simulink model "surveillance"  (Simulink 6.5)
settings: Solver=VariableStepDiscrete  StartTime=0.0  StopTime=inf  RelTol=1e-3
undefined symbols (not defined in the file or in its folder): gray
libraries: dspsnks4 x2, dspobslib x2, dspmtrx3 x2, dspsrcs4 x1, dspwin32 x1
settings Model: Creator=jacobf  LastModifiedBy=JacobF

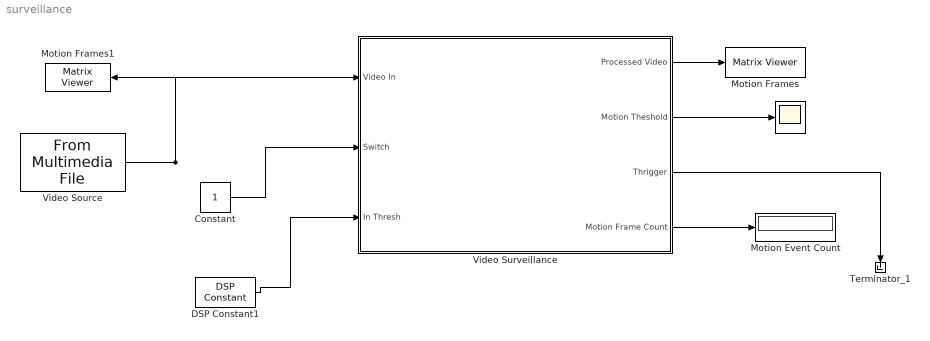
== system surveillance ==
  " " : Scope
      settings: TimeRange=18  YMin=0  YMax=500000
  Constant : Constant  Value=1  OutDataType=sfix(16)  ConRadixGroup=Use specified scaling  OutScaling=2^0  SampleTime=inf  FramePeriod=inf
  DSP Constant1 : dspsrcs4/DSP Constant  SystemSampleTime=-1  Value=1.5e5  SampleMode=Discrete  discreteOutput=Sample-based  continuousOutput=Sample-based  sampTime=1/15  framePeriod=2  dataType=int32  isSigned=on  wordLen=16  udDataType=sfix(16)  fracBitsMode=Best precision  numFracBits=15  InterpretAs1D=-inf  Ts=-inf  FramebasedOutput=-inf
      settings: additionalParams=on
  Motion Event Count : Display
  Motion Frames : dspsnks4/Matrix Viewer  DialogController=dspdialog.MatrixViewer  DialogControllerArgs=DataTag0  ImageParams=off  CMapStr=gray(256)  AxisColorbar=off  AxisParams=off  AxisOrigin=Upper left corner  XLabel=X-axis  YLabel=Y-axis  ZLabel=Z-axis  FigPos=[326 381 283 245]  AxisZoom=on
      settings: YMin=0  YMax=255
  Motion Frames1 : dspsnks4/Matrix Viewer  Orientation=left  DialogController=dspdialog.MatrixViewer  DialogControllerArgs=DataTag1  ImageParams=off  CMapStr=gray(256)  AxisColorbar=off  AxisParams=off  AxisOrigin=Upper left corner  XLabel=X-axis  YLabel=Y-axis  ZLabel=Z-axis  FigPos=[39 384 279 242]  AxisZoom=on
      settings: YMin=0  YMax=255
  Terminator_1 : Terminator
      settings: Orientation=down
  Video Source : dspwin32/From Multimedia File  DialogController=dspDDGCreate  DialogControllerArgs=DataTag2  inputFilename=vipmen.avi  loop=on  numPlays=inf  outputStreams=Video and audio  videoDataType=uint8  audioDataType=int16  inheritSampleTime=on  userDefinedSampleTime=1/30  noAudioOutput=off  isIntensityVideo=on  outputEOF=off
  "Video Surveillance " : Subsystem
  wires:
  Video Source/1 -> Motion Frames1/1, "Video Surveillance "/1(Video In)
  "Video Surveillance "/1(Processed Video) -> Motion Frames/1
  "Video Surveillance "/4(Motion Frame Count) -> Motion Event Count/1
  Constant/1 -> "Video Surveillance "/2(Switch)
  "Video Surveillance "/2(Motion Theshold) -> " "/1
  DSP Constant1/1 -> "Video Surveillance "/3(In Thresh)
  "Video Surveillance "/3(Thrigger) -> Terminator_1/1

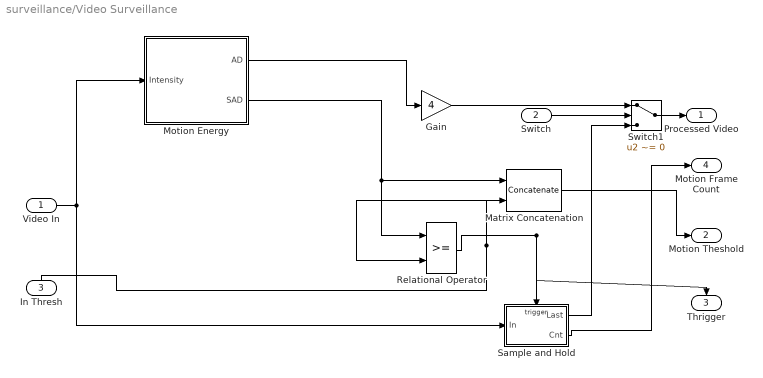
== system surveillance/Video Surveillance  ==
  Video In : Inport
  Switch : Inport  Port=2
  In Thresh : Inport  Orientation=up  Port=3
  Gain : Gain  Gain=4  ParameterDataType=uint(8)  OutDataTypeMode=Specify via dialog  OutDataType=uint(8)  SaturateOnIntegerOverflow=on
  Matrix Concatenation : Concatenate  Mode=Vertical matrix concatenation
  Motion Energy : Subsystem
  Relational Operator : RelationalOperator  LogicOutDataTypeMode=Boolean  InputSameDT=on
  Sample and Hold : Subsystem  AncestorBlock=dspsigops/Sample and Hold  TreatAsAtomicUnit=on  mask(Sample and Hold){trig=Either edge, initCond=0}
      mask prompts: trig "Trigger type:"; initCond "Initial condition:"
      mask help: Sample and hold input signal.
      mask init:
      | switch trig
      | case 1, s='rising';
      | case 2, s='falling';
      | case 3, s='either';
      | end
      | set_param([gcb '/Trigger'],'triggertype',s);
      mask Help: web(dspbhelp);
      mask StyleString: popup(Rising edge|Falling edge|Either edge),edit
      mask Display: disp('S/H')
  Switch1 : Switch  Criteria=u2 ~= 0  ZeroCross=off
  Processed Video : Outport
  Motion Theshold : Outport  Port=2
  Thrigger : Outport  Orientation=down  Port=3
  Motion Frame Count : Outport  Port=4
  wires:
  In Thresh/1 -> Relational Operator/2, Matrix Concatenation/2
  Motion Energy/1(AD) -> Gain/1
  Motion Energy/2(SAD) -> Matrix Concatenation/1, Relational Operator/1
  Gain/1 -> Switch1/1
  Sample and Hold/1(Last) -> Switch1/3
  Relational Operator/1 -> Sample and Hold/Trigger, Thrigger/1
  Video In/1 -> Motion Energy/1(Intensity), Sample and Hold/1(In)
  Switch/1 -> Switch1/2
  Switch1/1 -> Processed Video/1
  Matrix Concatenation/1 -> Motion Theshold/1
  Sample and Hold/2(" Cnt") -> Motion Frame Count/1

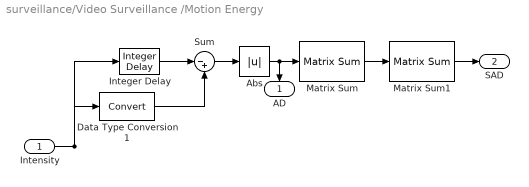
== system surveillance/Video Surveillance /Motion Energy ==
  Intensity : Inport
  Abs : Abs  SaturateOnIntegerOverflow=on  SampleTime=-1
  Data Type Conversion1 : DataTypeConversion  OutDataTypeMode=int16  RndMeth=Zero
  Integer Delay : dspobslib/Integer Delay  delay=1  ic=0  reset_popup=None
  Matrix Sum : dspmtrx3/Matrix Sum  DialogController=dspDDGCreate  DialogControllerArgs=DataTag3  Dim=Columns  outputMode=Binary point scaling  outputWordLength=32  outputFracLength=0  accumMode=Binary point scaling  accumWordLength=32  accumFracLength=0  roundingMode=Floor  overflowMode=off
      settings: additionalParams=on
  Matrix Sum1 : dspmtrx3/Matrix Sum  DialogController=dspDDGCreate  DialogControllerArgs=DataTag4  Dim=Rows  accumMode=Binary point scaling  accumWordLength=32  accumFracLength=0  roundingMode=Floor  overflowMode=off
  Sum : Sum  Inputs=|-+
  AD : Outport  Orientation=down
  SAD : Outport  Port=2
  wires:
  Sum/1 -> Abs/1
  Integer Delay/1 -> Sum/1
  Abs/1 -> Matrix Sum/1, AD/1
  Data Type Conversion1/1 -> Sum/2
  Matrix Sum/1 -> Matrix Sum1/1
  Intensity/1 -> Integer Delay/1, Data Type Conversion1/1
  Matrix Sum1/1 -> SAD/1

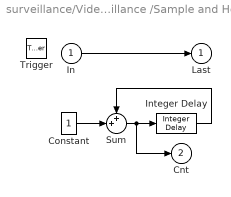
== system surveillance/Video Surveillance /Sample and Hold ==
  In : Inport
  Trigger : TriggerPort  TriggerType=either  StatesWhenEnabling=reset  ZeroCross=off
  Constant : Constant  Value=1  OutDataTypeMode=int32  OutDataType=sfix(16)  ConRadixGroup=Use specified scaling  OutScaling=2^0  SampleTime=inf  FramePeriod=inf
  Integer Delay : dspobslib/Integer Delay  delay=1  ic=0  reset_popup=None
  Sum : Sum  Inputs=++|
  Last : Outport  InitialOutput=initCond
  " Cnt" : Outport  Port=2
  wires:
  In/1 -> Last/1
  Constant/1 -> Sum/2
  Sum/1 -> Integer Delay/1, " Cnt"/1
  Integer Delay/1 -> Sum/1
